simulink model "ex2"  (R2020a)
settings: Solver=VariableStepAuto  StartTime=0.0  StopTime=10.0  RelTol=1e-3
settings Model: Creator=Kundan Patil  LastModifiedBy=Kundan Patil

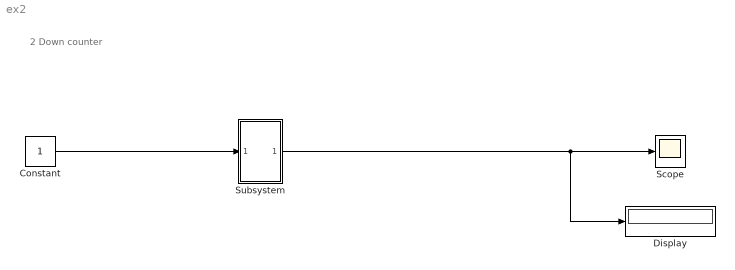
== system ex2 ==
  note: 2 Down counter
  Constant : Constant
  Display : Display
  Scope : Scope
  Subsystem : Subsystem
  wires:
  Subsystem/1(Out1) -> Display/1, Scope/1
  Constant/1 -> Subsystem/1(In1)

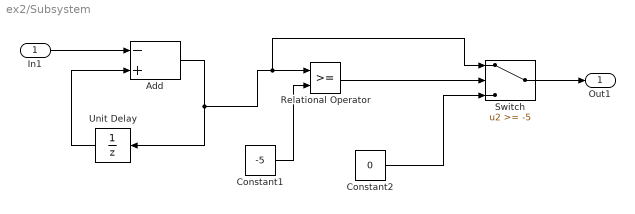
== system ex2/Subsystem ==
  In1 : Inport
  Add : Sum  Inputs=-+
  Constant1 : Constant  Value=-5
  Constant2 : Constant  Value=0
  Relational Operator : RelationalOperator  OutDataTypeStr=boolean  RndMeth=Simplest
  Switch : Switch  Threshold=-5
  Unit Delay : UnitDelay  InitialCondition=1  SampleTime=-1  HasFrameUpgradeWarning=on
  Out1 : Outport
  wires:
  Constant1/1 -> Relational Operator/2
  Add/1 -> Switch/1, Relational Operator/1, Unit Delay/1
  Relational Operator/1 -> Switch/2
  Switch/1 -> Out1/1
  Constant2/1 -> Switch/3
  Unit Delay/1 -> Add/2
  In1/1 -> Add/1
